simulink model "DDSCompiler_Ex1"  (R2025a)
settings: Solver=VariableStepDiscrete  StartTime=0.0  StopTime=1e6  RelTol=1e-3  EnableMultiTasking=on
libraries: hdlBasic x19, hdlDSPIP x1, hdlUtilities x1, dspsigops x1, vmcUtilities x1
settings Model: Creator=douangp  LastModifiedBy=robg
settings SolverCC: AlgebraicLoopSolver=TrustRegion
settings DataIOCC: LimitDataPoints=on  SaveFormat=Array  SignalLoggingSaveFormat=ModelDataLogs  ReturnWorkspaceOutputs=off
settings OptimizationCC: DefaultParameterBehavior=Inlined  ExpressionDepthLimit=2147483647.0  LifeSpan=inf
settings DebuggingCC: UnderspecifiedInitializationDetection=Classic  MergeDetectMultiDrivingBlocksExec=none  SolverPrmCheckMsg=warning  ParameterOverflowMsg=none  FcnCallInpInsideContextMsg=warning  UnconnectedInputMsg=warning  UnconnectedOutputMsg=warning  UnconnectedLineMsg=warning  AllowSymbolicDim=off  StateNameClashWarn=warning  SFUnexpectedBacktrackingDiag=warning  SFNoUnconditionalDefaultTransitionDiag=warning  SFExecutionAtInitializationDiag=none  ArithmeticOperatorsInVariantConditions=warning
settings HardwareCC: ProdBitPerPointer=32.0  ProdBitPerSizeT=32.0  ProdBitPerPtrDiffT=32.0  ProdLargestAtomicFloat=None  ProdIntDivRoundTo=Undefined  ProdEndianess=Unspecified  ProdWordSize=32.0  ProdHWDeviceType=32-bit Generic
settings ModelReferenceCC: EnableRefExpFcnMdlSchedulingChecks=on  PropagateSignalLabelsOutOfModel=off
settings SFSimCC: SimUseLocalCustomCode=off  CustomCodeUndefinedFunction=UseInterfaceOnly
settings RTWCC: RTWUseLocalCustomCode=off  GPUComputeCapability=3.5  DLArmComputeVersion=19.05
settings CodeAppCC: StateflowObjectComments=on
settings GRTTargetCC: TargetLangStandard=C89/C90 (ANSI)  CombineOutputUpdateFcns=off  GRTInterface=on
settings ConfigComp: CovMetricSettings=dw  CovSaveCumulativeToWorkspaceVar=on  CovSaveSingleToWorkspaceVar=on  CovExternalEMLEnable=off

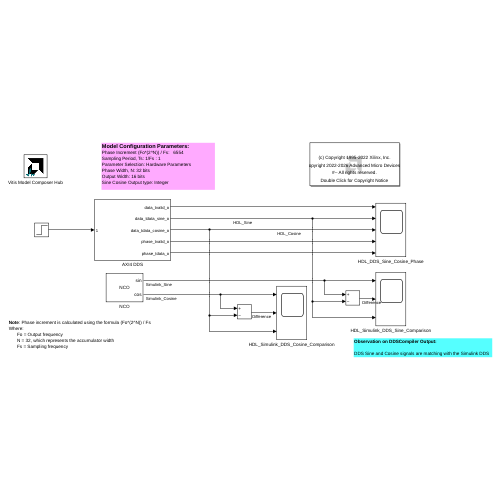
[thumbnail: Simulink's stored preview of the top-level diagram]
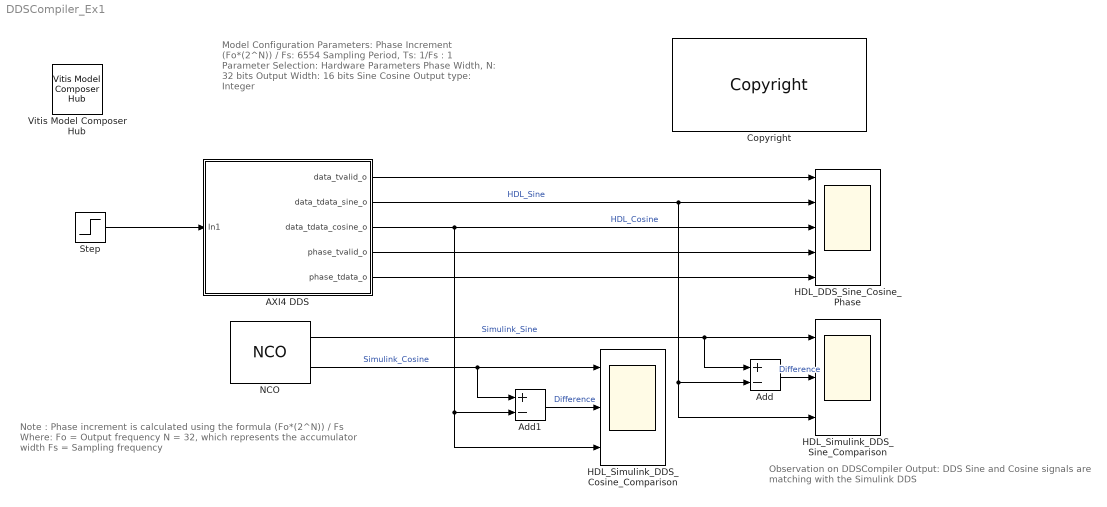
== system DDSCompiler_Ex1 ==
  note: Model Configuration Parameters:
      | Phase Increment (Fo*(2^N)) / Fs: 6554
      | Sampling Period, Ts: 1/Fs : 1
      | Parameter Selection: Hardware Parameters
      | Phase Width, N: 32 bits
      | Output Width: 16 bits
      | Sine Cosine Output type: Integer
  note: Note : Phase increment is calculated using the formula (Fo*(2^N)) / Fs
      | Where:
      | Fo = Output frequency
      | N = 32, which represents the accumulator width
      | Fs = Sampling frequency
  note: Observation on DDSCompiler Output:
      |
      | DDS Sine and Cosine signals are matching with the Simulink DDS
  AXI4 DDS : Subsystem
  Add : Sum  Inputs=+-
  Add1 : Sum  Inputs=+-
  Copyright : hdlUtilities/Copyright  copyrighttext="(c) Copyright 1995-2022 Xilinx, Inc. <br>(c) Copyright 2022-2026 Advanced Micro Devices, Inc. All rights reserved.<br><br>This document  contains proprietary, confidential information that may be used, copied and/or disclosed only as authorized by a valid licensing agreement with Advanced Micro Devices, Inc. This copyright notice must be retained on all authorized copies.<br><br> This code is provided \"as is\". Advanced Micro Devices, Inc. makes, and the end user receives, no warranties or conditions, express, implied, statutory or otherwise, and Advanced Micro Devices, Inc. specifically disclaims any implied warranties of merchantability, <br>non-infringement, or fitness for a particular purpose."  block_type=copyright
  HDL_DDS_Sine_Cosine_Phase : Scope  NumInputPorts=5
      settings: ActiveDisplayYMinimum=-0.125  ActiveDisplayYMaximum=1.125
  HDL_Simulink_DDS_Cosine_Comparison : Scope  NumInputPorts=3
      settings: ActiveDisplayYMinimum=-1  ActiveDisplayYMaximum=1  DataLoggingVariableName=ScopeData2
  HDL_Simulink_DDS_Sine_Comparison : Scope  NumInputPorts=3
      settings: ActiveDisplayYMinimum=-1  ActiveDisplayYMaximum=1
  NCO : dspsigops/NCO  AccIncSrc=Specify via dialog  AccInc=6554  PhaseOffsetSrc=Specify via dialog  PhaseOffset=0  AccumWL=32  HasDither=off  DitherWL=4  PNgeneratorLength=19  HasPhaseQuantizer=on  TableDepth=28  HasOutputPhaseError=off  Formula=Sine and cosine  DataType=Binary point scaling  OutputWL=16  OutputFL=15  CompMethod=Table lookup (no interpolation)  SampleTime=1  SamplesPerFrame=1  OutputFrames=off
  Step : Step  Time=5  SampleTime=0
  Vitis Model Composer Hub : vmcUtilities/Vitis Model Composer Hub  Tag=genX  CodeGeneration=off  SubsystemName=AXI4 DDS  StartColumn=1  NumberOfColumns=1  TargetDirectory=./code  exportDesign=off  analyzeDesign=off  validateDesignOnHw=off  ExportType=System Generator  IpVendor=xilinx.com  IpLibrary=hls  IpVersion=1.0  IpHWLanguage=Verilog  AieCompilerOptions={}  AieSimulatorOptions={}  CreateTestbench=off  TestbenchStackSize=10  RunRtlSim=off  RunCSim=off  RunAieSim=off  enableSimulationTimeout=on  enableGraphIterations=on  AieSimTimeout=50000  AieGraphIterations=-1  RunAieSimProfiling=off  LaunchVitisAnalyzer=off  PlotOutput=off  RunX86Sim=off  X86SimTimeout=10  GenHwImage=off  GenLibadfXo=on  GenHwValidationCode=off  PlatformType=Not Specified  HwSystemType=Baremetal  HwValidationTarget=hw  ProjDevice=xcku11p-ffva1156-1-e  ProjDevicePart=xcku11p-ffva1156-1-e  SamplePeriod=-1  ClockFrequency=200  DataPathParallelism=1  xilinxfamily=kintexuplus  part=xcku11p  speed=-1-e  package=ffva1156  directory=./netlist/ip/AXI4_DDS/src  testbench=off  incr_netlist=off  synthesis_tool=Vivado  clock_wrapper=Clock Enables  dbl_ovrd=According to Block Masks  dcm_input_clock_period=10  sysclk_period=10  simulink_period=1  eval_field=0  LogFileName=''  NThreads=4
  wires:
  Step/1 -> AXI4 DDS/1(In1)
  AXI4 DDS/1(data_tvalid_o) -> HDL_DDS_Sine_Cosine_Phase/1
  AXI4 DDS/2(data_tdata_sine_o) -> HDL_DDS_Sine_Cosine_Phase/2, Add/2, HDL_Simulink_DDS_Sine_Comparison/3  "HDL_Sine"
  AXI4 DDS/4(phase_tvalid_o) -> HDL_DDS_Sine_Cosine_Phase/4
  AXI4 DDS/5(phase_tdata_o) -> HDL_DDS_Sine_Cosine_Phase/5
  AXI4 DDS/3(data_tdata_cosine_o) -> HDL_DDS_Sine_Cosine_Phase/3, Add1/2, HDL_Simulink_DDS_Cosine_Comparison/3  "HDL_Cosine"
  NCO/1 -> Add/1, HDL_Simulink_DDS_Sine_Comparison/1  "Simulink_Sine"
  Add/1 -> HDL_Simulink_DDS_Sine_Comparison/2  "Difference"
  Add1/1 -> HDL_Simulink_DDS_Cosine_Comparison/2  "Difference"
  NCO/2 -> HDL_Simulink_DDS_Cosine_Comparison/1, Add1/1  "Simulink_Cosine"

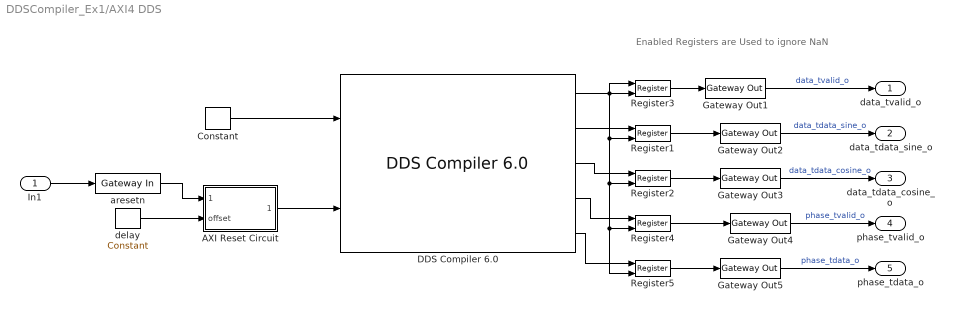
== system DDSCompiler_Ex1/AXI4 DDS ==
  note: Enabled Registers are Used to ignore NaN
  In1 : Inport
  AXI Reset Circuit : Subsystem
  Constant : hdlBasic/Constant  const=1  gui_display_data_type=Boolean  arith_type=Boolean  n_bits=16  bin_pt=14  preci_type=Single  exp_width=8  frac_width=24  explicit_period=on  period=1  XmcBlockStatus=1  maskContainerNames=tabcontainer1  block_type=constant  block_config=sysgen:Constant_config
  DDS Compiler 6.0 : hdlDSPIP/DDS Compiler 6.0   partspresent=Phase_Generator_and_SIN_COS_LUT  dds_clock_rate=100  channels=1  mode_of_operation=Standard  output_type=Integer  modulus=9  parameter_entry=Hardware_Parameters  spurious_free_dynamic_range=96.00000000  frequency_resolution=0.40000000  noise_shaping=None  phase_width=32  output_width=16  output_selection=Sine_and_Cosine  negative_sine=off  negative_cosine=off  amplitude_mode=Full_Range  memory_type=Auto  optimization_goal=Auto  dsp48_use=Minimal  resync=off  latency_configuration=Auto  latency=1  has_phase_out=on  has_aclken=off  has_aresetn=off  explicit_period=off  period=1  data_has_tlast=Not_Required  has_tready=on  s_phase_has_tuser=Not_Required  m_data_has_tuser=Not_Required  m_phase_has_tuser=Not_Required  s_phase_tuser_width=1  output_form=Twos_Complement  s_config_sync_mode=On_Vector  phase_increment=Fixed  output_frequency1=0  output_frequency2=0  output_frequency3=0  output_frequency4=0  output_frequency5=0  output_frequency6=0  output_frequency7=0  output_frequency8=0  output_frequency9=0  output_frequency10=0  output_frequency11=0  output_frequency12=0  output_frequency13=0  output_frequency14=0  output_frequency15=0  output_frequency16=0  pinc1=dec2bin(6554)  pinc2='0'  pinc3='0'  pinc4='0'  pinc5='0'  pinc6='0'  pinc7='0'  pinc8='0'  pinc9='0'  pinc10='0'  pinc11='0'  pinc12='0'  pinc13='0'  pinc14='0'  pinc15='0'  pinc16='0'  phase_offset=None  phase_offset_angles1=0  phase_offset_angles2=0  phase_offset_angles3=0  phase_offset_angles4=0  phase_offset_angles5=0  phase_offset_angles6=0  phase_offset_angles7=0  phase_offset_angles8=0  phase_offset_angles9=0  phase_offset_angles10=0  phase_offset_angles11=0  phase_offset_angles12=0  phase_offset_angles13=0  phase_offset_angles14=0  phase_offset_angles15=0  phase_offset_angles16=0  poff1='0'  poff2='0'  poff3='0'  poff4='0'  poff5='0'  poff6='0'  poff7='0'  poff8='0'  poff9='0'  poff10='0'  poff11='0'  poff12='0'  poff13='0'  poff14='0'  poff15='0'  poff16='0'  trim_axipin_name=on  simulation_type=hybrid_sim  simulation_model=sysgen:xddsv6_0_cmodel  data_path_portlist={ 's_axis_config_tdata_poff', 's_axis_config_tdata_chan0_poff', 's_axis_config_tdata_pinc', 's_axis_config_tdata_chan0_pinc', 's_axis_phase_tdata_resync', 's_axis_phase_tdata_chan0_resync', 's_axis_phase_tdata_poff', 's_axis_phase_tdata_chan0_poff', 's_axis_phase_tdata_pinc', 's_axis_phase_tdata_chan0_pinc', 's_axis_phase_tdata_phase_in', 'm_axis_data_tdata_sine', 'm_axis_data_tdata_chan0_sine', 'm_axis_data_tdata_cosine', 'm_axis_data_tdata_chan0_cosine', 'm_axis_phase_tdata_phase_out', 'm_axis_phase_tdata_chan0_phase_out'}  por_mode=false  gui_behaviour=Sysgen  ip_name=DDS Compiler  ip_version=6.0  dsptool_ready=true  wrapper_available=true  port_translation_map={ 'aclken' => 'en', 'aresetn' => 'rst' }  ipcore_usecache=true  ipcore_useipmodelcache=true  ipcore_xco_need_fpga_part=true  ipcore_fpga_part=[]  ipcore_verbose=false  XmcBlockStatus=1  maskContainerNames=tabcontainer1  block_type=dds_compiler_v6_0  block_config=sysgen:rodinimport_config  block_width=760
  Gateway Out{1..5} (5 alike) : hdlBasic/Gateway Out  inherit_from_input=on  bool_to_boolean=off  hdl_port=on  rows=1  columns=1  UseAsDAC=off  DACChannel='1'  interface=None  automatic_assignment=on  address_offset=hex2dec('00')  intf_name=''  intf_description=''  timing_constraint=None  locs_specified=off  LOCs={}  io_standard={}  XmcBlockStatus=1  maskContainerNames=group4  block_type=gatewayout  block_config=sysgen:gateway_out_config  block_width_w=590  block_height_w=620  block_width=620  block_height=750
  Register{1..5} (5 alike) : hdlBasic/Register  init=0  rst=off  en=on  XmcBlockStatus=1  maskContainerNames=tabcontainer1  block_type=register  block_config=sysgen:Register_config
  aresetn : hdlBasic/Gateway In  gui_display_data_type=Boolean  arith_type=Boolean  n_bits=1  bin_pt=0  preci_type=Single  exp_width=8  frac_width=24  rows=1  columns=1  quantization="Round  (unbiased: +/- Inf)"  overflow=Saturate  period=1  UseAsADC=off  ADCChannel='1'  interface=None  automatic_assignment=on  address_offset=hex2dec('00')  intf_name=''  intf_description=''  default_value=0  timing_constraint=None  locs_specified=off  LOCs={}  io_standard={}  inherit_from_input=off  hdl_port=on  XmcBlockStatus=1  maskContainerNames=group4  block_type=gatewayin  block_config=sysgen:gateway_in_config  block_width_w=590  block_height_w=620  block_width=640  block_height=850
  delay : hdlBasic/Constant  const=10  gui_display_data_type=Fixed-point  arith_type=Unsigned  n_bits=8  bin_pt=0  preci_type=Single  exp_width=8  frac_width=24  explicit_period=off  period=1  XmcBlockStatus=1  maskContainerNames=tabcontainer1  block_type=constant  block_config=sysgen:Constant_config
  data_tvalid_o : Outport
  data_tdata_sine_o : Outport  Port=2
  data_tdata_cosine_o : Outport  Port=3
  phase_tvalid_o : Outport  Port=4
  phase_tdata_o : Outport  Port=5
  wires:
  In1/1 -> aresetn/1
  Constant/1 -> DDS Compiler 6.0/1
  AXI Reset Circuit/1(valid_out) -> DDS Compiler 6.0/2
  Register1/1 -> Gateway Out2/1
  DDS Compiler 6.0/2 -> Register1/1
  Register2/1 -> Gateway Out3/1
  Gateway Out3/1 -> data_tdata_cosine_o/1  "data_tdata_cosine_o"
  Gateway Out2/1 -> data_tdata_sine_o/1  "data_tdata_sine_o"
  Gateway Out1/1 -> data_tvalid_o/1  "data_tvalid_o"
  aresetn/1 -> AXI Reset Circuit/1(valid_in)
  delay/1 -> AXI Reset Circuit/2(offset)
  Register3/1 -> Gateway Out1/1
  DDS Compiler 6.0/3 -> Register2/1
  Gateway Out4/1 -> phase_tvalid_o/1  "phase_tvalid_o"
  DDS Compiler 6.0/1 -> Register3/2, Register3/1, Register1/2, Register5/2, Register4/2, Register2/2
  Register4/1 -> Gateway Out4/1
  Gateway Out5/1 -> phase_tdata_o/1  "phase_tdata_o"
  Register5/1 -> Gateway Out5/1
  DDS Compiler 6.0/4 -> Register4/1
  DDS Compiler 6.0/5 -> Register5/1

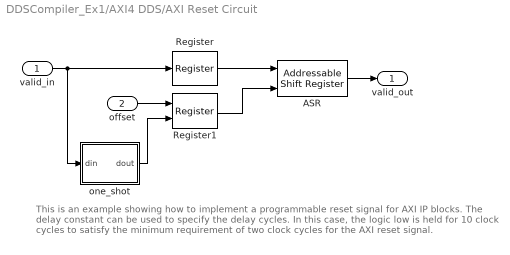
== system DDSCompiler_Ex1/AXI4 DDS/AXI Reset Circuit ==
  note: This is an example showing how to implement a programmable reset signal
      |  for AXI IP blocks. The delay constant can be used to specify the delay cycles.
      | In this case, the logic low is held for 10 clock cycles to satisfy the minimum
      | requirement of two clock cycles for the AXI reset signal.
  valid_in : Inport
  offset : Inport  Port=2
  ASR : hdlBasic/Addressable Shift Register  infer_latency=on  depth=2  initVector=[0]  en=off  use_behavioral_HDL=off  Optimization=Resource  use_rpm=on  XmcBlockStatus=1  maskContainerNames=group1  block_type=addrsr  block_config=sysgen:Addrsr_config
  Register : hdlBasic/Register  init=0  rst=off  en=off  XmcBlockStatus=1  maskContainerNames=tabcontainer1  block_type=register  block_config=sysgen:Register_config
  Register1 : hdlBasic/Register  init=0  rst=off  en=on  XmcBlockStatus=1  maskContainerNames=tabcontainer1  block_type=register  block_config=sysgen:Register_config
  one_shot : Subsystem
  valid_out : Outport  VectorParamsAs1DForOutWhenUnconnected=off
  wires:
  valid_in/1 -> Register/1, one_shot/1(din)
  Register/1 -> ASR/1
  ASR/1 -> valid_out/1
  Register1/1 -> ASR/2
  offset/1 -> Register1/1
  one_shot/1(dout) -> Register1/2

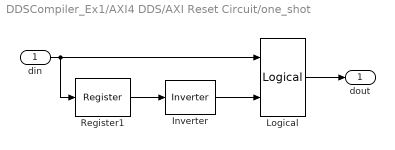
== system DDSCompiler_Ex1/AXI4 DDS/AXI Reset Circuit/one_shot ==
  din : Inport
  Inverter : hdlBasic/Inverter  en=off  latency=0  XmcBlockStatus=1  maskContainerNames=group2  block_type=inv  block_config=sysgen:Inverter_config
  Logical : hdlBasic/Logical  logical_function=AND  inputs=2  en=off  latency=0  precision=Full  arith_type=Unsigned  n_bits=8  bin_pt=2  align_bp=on  overflow=[]  quantization=[]  XmcBlockStatus=1  maskContainerNames=tabcontainer1  block_type=logical  block_config=sysgen:Logical_config
  Register1 : hdlBasic/Register  init=0  rst=off  en=off  XmcBlockStatus=1  maskContainerNames=tabcontainer1  block_type=register  block_config=sysgen:Register_config
  dout : Outport  VectorParamsAs1DForOutWhenUnconnected=off
  wires:
  din/1 -> Logical/1, Register1/1
  Register1/1 -> Inverter/1
  Inverter/1 -> Logical/2
  Logical/1 -> dout/1
